simulink model "identificationV1"  (R2023b)
settings: Solver=VariableStepAuto  StartTime=0.0  StopTime=10.0  FixedStep=0.0066666666666666671  MaxStep=0.1e-3
values from neighbouring files (symbols this model uses):
  AMPLITUDE = 100    [params.m]
  FREQUENCY = 2*pi*50    (= 314.159265359)    [params.m]
undefined symbols (not defined in the file or in its folder): Noise
libraries: simulink x1
settings Model: Creator=gosmann  LastModifiedBy=meneu
settings SolverCC: MaxConsecutiveMinStep=100

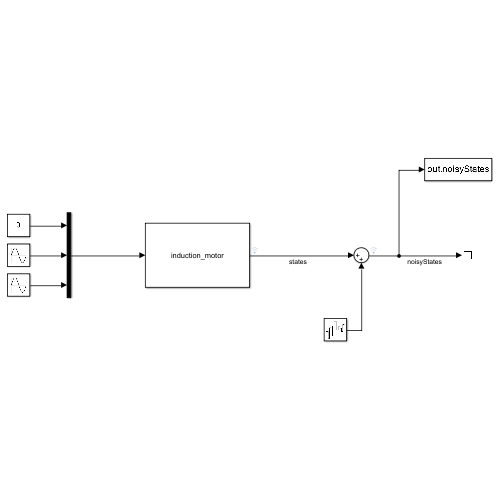
[thumbnail: Simulink's stored preview of the top-level diagram]
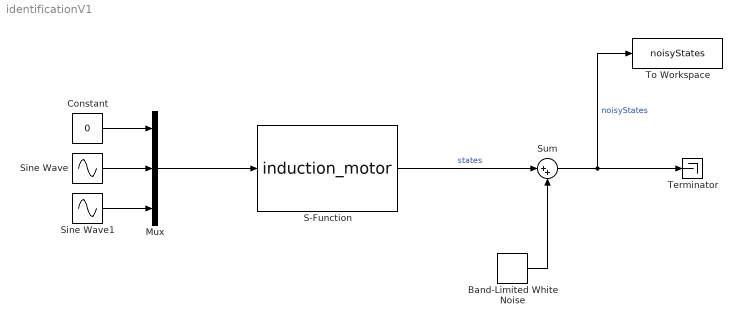
== system identificationV1 ==
  Band-Limited White Noise : simulink/Sources/Band-Limited White Noise  Cov=[Noise.power]  Ts=Noise.sampleTime  seed=[23341]
  Constant : Constant  Value=0
  Mux : Mux  Inputs=3
  S-Function : S-Function  FunctionName=induction_motor  Parameters=parameters  SFunctionDeploymentMode=off  EnableBusSupport=off
  Sine Wave : Sin  Amplitude=AMPLITUDE  Frequency=FREQUENCY  SampleTime=0
  Sine Wave1 : Sin  Amplitude=AMPLITUDE  Frequency=FREQUENCY  Phase=0-(pi/180)*90  SampleTime=0
  Sum : Sum  Inputs=|++
  Terminator : Terminator
  To Workspace : ToWorkspace  VariableName=noisyStates  SaveFormat=Timeseries  SampleTime=-1
  wires:
  Mux/1 -> S-Function/1
  Sine Wave1/1 -> Mux/3
  Sine Wave/1 -> Mux/2
  Constant/1 -> Mux/1
  Sum/1 -> To Workspace/1, Terminator/1  "noisyStates"
  S-Function/1 -> Sum/1  "states"
  Band-Limited White Noise/1 -> Sum/2
